simulink library "Healthcare_Center_Department"  (R2019a)
settings: Solver=VariableStepAuto  StartTime=0.0  StopTime=10.0  RelTol=1e-3
undefined symbols (not defined in the file or in its folder): m, n
settings Model: Creator=arsineh  LastModifiedBy=arsineh

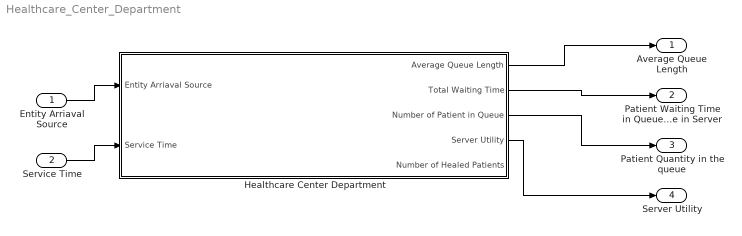
== system Healthcare_Center_Department ==
  Entity Arriaval Source : Inport
  Service Time : Inport  Port=2
  Healthcare Center Department : Subsystem
  Average Queue Length : Outport
  "Patient Waiting Time in Queue + Patient Examination Time in Server " : Outport  Port=2
  Patient Quantity in the queue : Outport  Port=3
  Server Utility : Outport  Port=4
  wires:
  Entity Arriaval Source/1 -> Healthcare Center Department/1(Entity Arriaval Source)
  Healthcare Center Department/3(Number of Patient in Queue) -> Patient Quantity in the queue/1
  Service Time/1 -> Healthcare Center Department/2(Service Time)
  Healthcare Center Department/1(Average Queue Length) -> Average Queue Length/1
  Healthcare Center Department/2(Total Waiting Time) -> "Patient Waiting Time in Queue + Patient Examination Time in Server "/1
  Healthcare Center Department/4(Server Utility) -> Server Utility/1

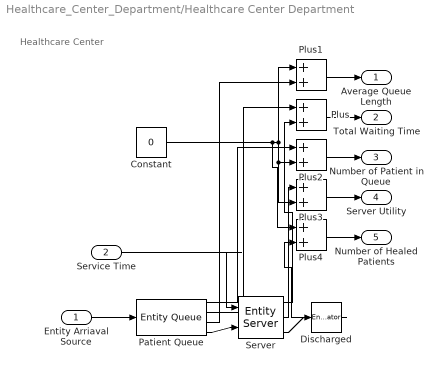
== system Healthcare_Center_Department/Healthcare Center Department ==
  note: Healthcare Center
  Entity Arriaval Source : Inport
  Service Time : Inport  Port=2
  Constant : Constant  Value=0
  Discharged : EntityTerminator  InputPortMessageModes=m  NumberEntitiesArrived=on
      settings: OutputPortMap=o0
  Patient Queue : EntityQueue  InputPortMessageModes=m  OutputPortMessageModes=n,n,n,m  Capacity=100000  NumberEntitiesInBlock=on  AverageWait=on  AverageQueueLength=on
      settings: OutputPortMap=o1,o2,o3,o5
  Plus{,1..4} (5 alike) : Sum
  Server : EntityServer  InputPortMessageModes=n,m  OutputPortMessageModes=n,n,m  Capacity=4000  ServiceTimeSource=Signal port  AverageWait=on  Utilization=on
      settings: InputPortMap=u0,u2  OutputPortMap=o4,o5,o9
  Average Queue Length : Outport
  Total Waiting Time : Outport  Port=2
  Number of Patient in Queue : Outport  Port=3
  Server Utility : Outport  Port=4
  Number of Healed Patients : Outport  Port=5
  wires:
  Patient Queue/4 -> Server/2
  Entity Arriaval Source/1 -> Patient Queue/1
  Patient Queue/1 -> Plus2/1
  Service Time/1 -> Server/1
  Patient Queue/3 -> Plus1/2
  Plus/1 -> Total Waiting Time/1
  Patient Queue/2 -> Plus/1
  Server/1 -> Plus/2
  Server/2 -> Plus3/1
  Server/3 -> Discharged/1
  Constant/1 -> Plus4/1, Plus1/1, Plus3/2, Plus2/2
  Plus1/1 -> Average Queue Length/1
  Plus2/1 -> Number of Patient in Queue/1
  Plus3/1 -> Server Utility/1
  Discharged/1 -> Plus4/2
  Plus4/1 -> Number of Healed Patients/1
